simulink model "ES005A_TmplMonr"  (R2013b)
settings: Solver=FixedStepDiscrete  SolverMode=SingleTasking  StartTime=0.0  StopTime=1  FixedStep=0.002  RelTol=1e-3
undefined symbols (not defined in the file): ELECGLBPRM_STRTUPSTDI_CNT_U08, ELECGLBPRM_STRTUPSTTMPLMONININTESTSTRT_CNT_U08, IninFlt, RtFlt, SpiConf_SpiChannel_TmplMonrCh1, SpiConf_SpiChannel_TmplMonrCh2, SpiConf_SpiChannel_TmplMonrCh3, SpiConf_SpiSequence_TmplMonrSeq1, SpiConf_SpiSequence_TmplMonrSeq2, SpiConf_SpiSequence_TmplMonrSeq3, STD_HIGH, STD_LOW, TMPLMONRCFGREG1READVAL_CNT_U16, TMPLMONRCFGREG1WRVAL_CNT_U16, TMPLMONRSTSREG2READVAL_CNT_U16, TMPLMONRWDGMODKEYWORD1_CNT_U16, TMPLMONRWDGMODKEYWORD2_CNT_U16, TMPLMONRWDGMODKEYWORD3_CNT_U16, TrigReg1
libraries: simulink x12
(part 2 of 4)

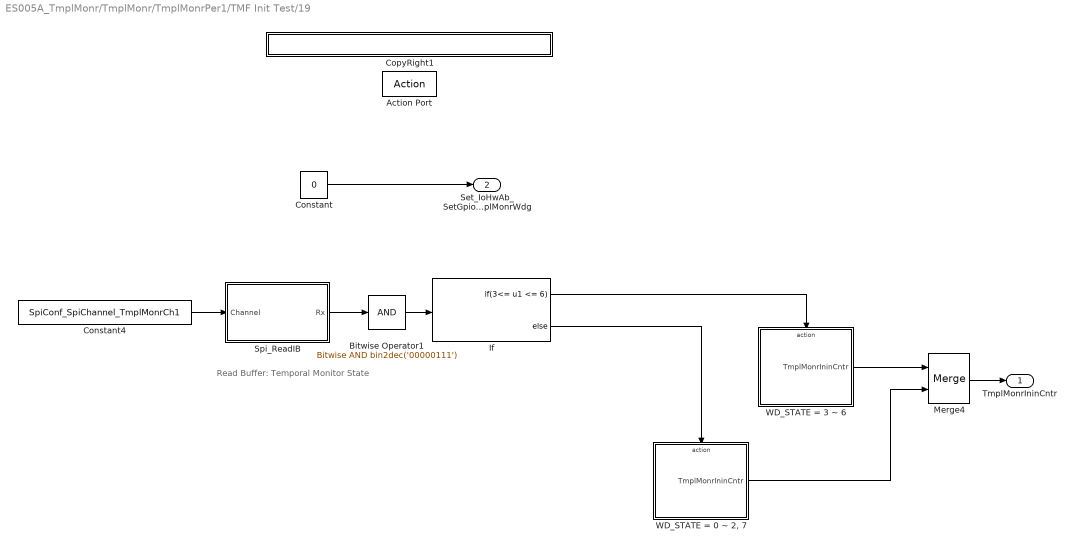
== system ES005A_TmplMonr/TmplMonr/TmplMonrPer1/TMF Init Test/19 ==
  note: Read Buffer: Temporal Monitor State
  Action Port : ActionPort  ActionType=case
  Bitwise Operator1 : simulink/Logic and Bit Operations/Bitwise Operator  logicop=AND  UseBitMask=on  BitMask=bin2dec('00000111')  BitMaskRealWorld=Stored Integer
  Constant : Constant  Value=0  OutDataTypeStr=boolean
  Constant4 : Constant  Value=SpiConf_SpiChannel_TmplMonrCh1  OutDataTypeStr=uint8
  CopyRight1 : Subsystem  Description=|  mask(Copyright Information){none=on}
      | Copyright info block.                                               
      |                                                                     
      | Place copyright information at the top of every subsystem in design.
      mask prompts: none "No parameters"
      mask help: Place copyright information at the top of every subsystem in design.
      mask Display:
      | NxtrConf = 'Nexteer Confidential';
      | 
      | sys = bdroot; %handle for the current model ("system")
      | first = get_param(sys,'Created');
      | first = first(end-3:end);  %year is last four digits
      | 
      | last = get_param(sys,'LastModifiedDate');
      | if isempty(last)
      |     last = datestr(now,'yyyy');
      | else
      |     last = last(end-3:end);
      | end
      | 
      | if strcmp(first,last)
      |     fprintf('%s -- Copyright %s Nexteer',NxtrConf,first)
      | else
      |     fprintf('%s -- %s%s- %s Nexteer',NxtrConf,char(169),first,last)
      | end
  If : If  IfExpression=3<= u1 <= 6
  Merge4 : Merge
  Spi_ReadIB : Subsystem
  "WD_STATE = 0 ~ 2, 7" : Subsystem  RequirementInfo="{'linktype_rmi_doors' '0000c46a (/ESG Group/FDD Module Requirements/EA4 Specific/ES005A_TmplMonr)' '#ES005A_177' 'true' 'REQ: ES005A_177' '' ; 'linktype_rmi_doors' '0000c46a (/ESG Group/FDD Module Requirements/EA4 Specific/ES005A_TmplMonr)' '#ES005A_182' 'true' 'REQ:  ES005A_182' '' } %GIDa_08cc5124_a215_4196_a476_7ca0c813cfd0"
  WD_STATE = 3 ~ 6 : Subsystem
  TmplMonrIninCntr : Outport
  Set_IoHwAb_SetGpioTmplMonrWdg : Outport  Port=2
  wires:
  Bitwise Operator1/1 -> If/1
  If/1 -> WD_STATE = 3 ~ 6/Action
  Constant4/1 -> Spi_ReadIB/1(Channel)
  Spi_ReadIB/1(Rx) -> Bitwise Operator1/1
  If/2 -> "WD_STATE = 0 ~ 2, 7"/Action
  Constant/1 -> Set_IoHwAb_SetGpioTmplMonrWdg/1
  WD_STATE = 3 ~ 6/1(TmplMonrIninCntr) -> Merge4/1
  "WD_STATE = 0 ~ 2, 7"/1(TmplMonrIninCntr) -> Merge4/2
  Merge4/1 -> TmplMonrIninCntr/1

== system ES005A_TmplMonr/TmplMonr/TmplMonrPer1/TMF Init Test/20 ==
  note: 1
  note: Read Cmd: Edge, Valid - 10010000000000
  Action Port : ActionPort  ActionType=case
  Call_Spi_AsyncTransmit : Subsystem
  Constant : Constant  Value=0  OutDataTypeStr=boolean
  Constant2 : Constant  OutDataTypeStr=uint8
  Constant4 : Constant  Value=SpiConf_SpiSequence_TmplMonrSeq3  OutDataTypeStr=uint8
  Constant5 : Constant  Value=SpiConf_SpiChannel_TmplMonrCh3  OutDataTypeStr=uint8
  Constant6 : Constant  Value=TMPLMONRCFGREG1READVAL_CNT_U16  OutDataTypeStr=uint16
  CopyRight1 : Subsystem  Description=|  mask(Copyright Information){none=on}
      | Copyright info block.                                               
      |                                                                     
      | Place copyright information at the top of every subsystem in design.
      mask prompts: none "No parameters"
      mask help: Place copyright information at the top of every subsystem in design.
      mask Display:
      | NxtrConf = 'Nexteer Confidential';
      | 
      | sys = bdroot; %handle for the current model ("system")
      | first = get_param(sys,'Created');
      | first = first(end-3:end);  %year is last four digits
      | 
      | last = get_param(sys,'LastModifiedDate');
      | if isempty(last)
      |     last = datestr(now,'yyyy');
      | else
      |     last = last(end-3:end);
      | end
      | 
      | if strcmp(first,last)
      |     fprintf('%s -- Copyright %s Nexteer',NxtrConf,first)
      | else
      |     fprintf('%s -- %s%s- %s Nexteer',NxtrConf,char(169),first,last)
      | end
  Spi_WriteIB : Subsystem
  TmplMonrIninCntr : Outport
  Set_IoHwAb_SetGpioTmplMonrWdg : Outport  Port=2
  wires:
  Constant2/1 -> TmplMonrIninCntr/1
  Constant4/1 -> Call_Spi_AsyncTransmit/1(Sequence)
  Constant5/1 -> Spi_WriteIB/1(Channel)
  Constant6/1 -> Spi_WriteIB/2(DataBufferPtr)
  Constant/1 -> Set_IoHwAb_SetGpioTmplMonrWdg/1

== system ES005A_TmplMonr/TmplMonr/TmplMonrPer1/TMF Init Test/21 ==
  note: In normal condition the value should be
      | BIN=1011 DEC=11
  note: Read Buffer: Edge/Valid
  Action Port : ActionPort  ActionType=case
  Bitwise Operator1 : simulink/Logic and Bit Operations/Bitwise Operator  logicop=AND  UseBitMask=on  BitMask=bin2dec('00001111')  BitMaskRealWorld=Stored Integer
  Constant : Constant  Value=0  OutDataTypeStr=boolean
  Constant2 : Constant  OutDataTypeStr=uint8
  Constant4 : Constant  Value=SpiConf_SpiChannel_TmplMonrCh3  OutDataTypeStr=uint8
  CopyRight1 : Subsystem  Description=|  mask(Copyright Information){none=on}
      | Copyright info block.                                               
      |                                                                     
      | Place copyright information at the top of every subsystem in design.
      mask prompts: none "No parameters"
      mask help: Place copyright information at the top of every subsystem in design.
      mask Display:
      | NxtrConf = 'Nexteer Confidential';
      | 
      | sys = bdroot; %handle for the current model ("system")
      | first = get_param(sys,'Created');
      | first = first(end-3:end);  %year is last four digits
      | 
      | last = get_param(sys,'LastModifiedDate');
      | if isempty(last)
      |     last = datestr(now,'yyyy');
      | else
      |     last = last(end-3:end);
      | end
      | 
      | if strcmp(first,last)
      |     fprintf('%s -- Copyright %s Nexteer',NxtrConf,first)
      | else
      |     fprintf('%s -- %s%s- %s Nexteer',NxtrConf,char(169),first,last)
      | end
  Edge/Valid Cnts are NOT Correct : Subsystem  RequirementInfo={'linktype_rmi_doors' '0000c46a (/ESG Group/FDD Module Requirements/EA4 Specific/ES005A_TmplMonr)' '#ES005A_176' 'true' 'REQ: ES005A_176' '' } %GIDa_dd7b43f1_2995_4ab0_82fe_3b40abf5c3b8
  If : If  IfExpression=u1 ~= 11  ShowElse=off
  Spi_ReadIB : Subsystem
  TmplMonrIninCntr : Outport
  Set_IoHwAb_SetGpioTmplMonrWdg : Outport  Port=2
  wires:
  Constant4/1 -> Spi_ReadIB/1(Channel)
  Spi_ReadIB/1(Rx) -> Bitwise Operator1/1
  Bitwise Operator1/1 -> If/1
  If/1 -> Edge/Valid Cnts are NOT Correct/Action
  Constant/1 -> Set_IoHwAb_SetGpioTmplMonrWdg/1
  Constant2/1 -> TmplMonrIninCntr/1

== system ES005A_TmplMonr/TmplMonr/TmplMonrPer1/TMF Init Test/22-52 ==
  Action Port : ActionPort  ActionType=case
  Constant : Constant  OutDataTypeStr=boolean
  Constant2 : Constant  OutDataTypeStr=uint8
  CopyRight1 : Subsystem  Description=|  mask(Copyright Information){none=on}
      | Copyright info block.                                               
      |                                                                     
      | Place copyright information at the top of every subsystem in design.
      mask prompts: none "No parameters"
      mask help: Place copyright information at the top of every subsystem in design.
      mask Display:
      | NxtrConf = 'Nexteer Confidential';
      | 
      | sys = bdroot; %handle for the current model ("system")
      | first = get_param(sys,'Created');
      | first = first(end-3:end);  %year is last four digits
      | 
      | last = get_param(sys,'LastModifiedDate');
      | if isempty(last)
      |     last = datestr(now,'yyyy');
      | else
      |     last = last(end-3:end);
      | end
      | 
      | if strcmp(first,last)
      |     fprintf('%s -- Copyright %s Nexteer',NxtrConf,first)
      | else
      |     fprintf('%s -- %s%s- %s Nexteer',NxtrConf,char(169),first,last)
      | end
  TmplMonrIninCntr : Outport
  Set_IoHwAb_SetGpioTmplMonrWdg : Outport  Port=2
  wires:
  Constant2/1 -> TmplMonrIninCntr/1
  Constant/1 -> Set_IoHwAb_SetGpioTmplMonrWdg/1

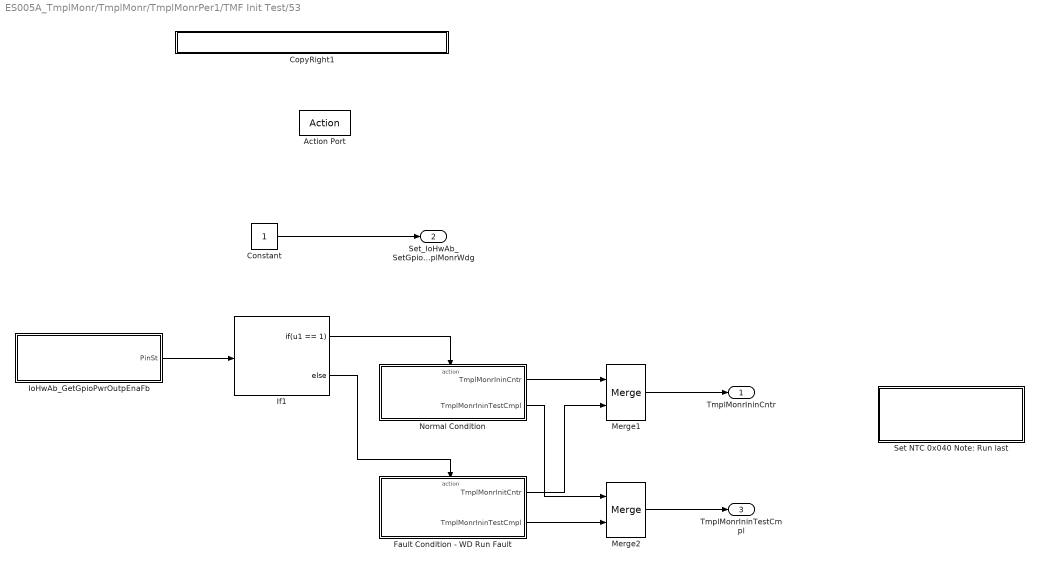
== system ES005A_TmplMonr/TmplMonr/TmplMonrPer1/TMF Init Test/53 ==
  Action Port : ActionPort  ActionType=case
  Constant : Constant  OutDataTypeStr=boolean
  CopyRight1 : Subsystem  Description=|  mask(Copyright Information){none=on}
      | Copyright info block.                                               
      |                                                                     
      | Place copyright information at the top of every subsystem in design.
      mask prompts: none "No parameters"
      mask help: Place copyright information at the top of every subsystem in design.
      mask Display:
      | NxtrConf = 'Nexteer Confidential';
      | 
      | sys = bdroot; %handle for the current model ("system")
      | first = get_param(sys,'Created');
      | first = first(end-3:end);  %year is last four digits
      | 
      | last = get_param(sys,'LastModifiedDate');
      | if isempty(last)
      |     last = datestr(now,'yyyy');
      | else
      |     last = last(end-3:end);
      | end
      | 
      | if strcmp(first,last)
      |     fprintf('%s -- Copyright %s Nexteer',NxtrConf,first)
      | else
      |     fprintf('%s -- %s%s- %s Nexteer',NxtrConf,char(169),first,last)
      | end
  Fault Condition - WD Run Fault : Subsystem  RequirementInfo={} %GIDa_b93698f8_2763_40bb_9d1b_225acd7973d3
  If1 : If  IfExpression=u1 == 1
  IoHwAb_GetGpioPwrOutpEnaFb : Subsystem
  Merge1 : Merge
  Merge2 : Merge
  Normal Condition : Subsystem  RequirementInfo={'linktype_rmi_doors' '0000c46a (/ESG Group/FDD Module Requirements/EA4 Specific/ES005A_TmplMonr)' '#ES005A_164' 'true' 'REQ: ES005A_164' '' } %GIDa_785a744b_ba8b_461e_b98b_5c61c0bc0772
  Set NTC 0x040 Note: Run last : Subsystem  RequirementInfo="{'linktype_rmi_doors' '0000c46a (/ESG Group/FDD Module Requirements/EA4 Specific/ES005A_TmplMonr)' '#ES005A_183' 'true' 'REQ:  ES005A_183' '' } %GIDa_d81dec6a_41a1_4ea0_a985_1fcdbb0d2b96"
  TmplMonrIninCntr : Outport
  Set_IoHwAb_SetGpioTmplMonrWdg : Outport  Port=2
  TmplMonrIninTestCmpl : Outport  Port=3
  wires:
  If1/1 -> Normal Condition/Action
  If1/2 -> Fault Condition - WD Run Fault/Action
  IoHwAb_GetGpioPwrOutpEnaFb/1(PinSt) -> If1/1
  Normal Condition/1(TmplMonrIninCntr) -> Merge1/1
  Fault Condition - WD Run Fault/1(TmplMonrInitCntr) -> Merge1/2
  Constant/1 -> Set_IoHwAb_SetGpioTmplMonrWdg/1
  Merge1/1 -> TmplMonrIninCntr/1
  Merge2/1 -> TmplMonrIninTestCmpl/1
  Normal Condition/2(TmplMonrIninTestCmpl) -> Merge2/1
  Fault Condition - WD Run Fault/2(TmplMonrIninTestCmpl) -> Merge2/2

== system ES005A_TmplMonr/TmplMonr/TmplMonrPer1/TMF Init Test/CopyRight1 ==

== system ES005A_TmplMonr/TmplMonr/TmplMonrPer1/TMF Init Test/Default ==
  note: DO NOTHING
  Action Port : ActionPort  ActionType=default
  CopyRight1 : Subsystem  Description=|  mask(Copyright Information){none=on}
      | Copyright info block.                                               
      |                                                                     
      | Place copyright information at the top of every subsystem in design.
      mask prompts: none "No parameters"
      mask help: Place copyright information at the top of every subsystem in design.
      mask Display:
      | NxtrConf = 'Nexteer Confidential';
      | 
      | sys = bdroot; %handle for the current model ("system")
      | first = get_param(sys,'Created');
      | first = first(end-3:end);  %year is last four digits
      | 
      | last = get_param(sys,'LastModifiedDate');
      | if isempty(last)
      |     last = datestr(now,'yyyy');
      | else
      |     last = last(end-3:end);
      | end
      | 
      | if strcmp(first,last)
      |     fprintf('%s -- Copyright %s Nexteer',NxtrConf,first)
      | else
      |     fprintf('%s -- %s%s- %s Nexteer',NxtrConf,char(169),first,last)
      | end

== system ES005A_TmplMonr/TmplMonr/TmplMonrPer1/TMF Init Test/IoHwAb_SetGpioTmplMonrWdg ==
  Trigger : TriggerPort  PortDimensions=1
  Constant1 : Constant  OutDataTypeStr=boolean
  CopyRight1 : Subsystem  Description=|  mask(Copyright Information){none=on}
      | Copyright info block.                                               
      |                                                                     
      | Place copyright information at the top of every subsystem in design.
      mask prompts: none "No parameters"
      mask help: Place copyright information at the top of every subsystem in design.
      mask Display:
      | NxtrConf = 'Nexteer Confidential';
      | 
      | sys = bdroot; %handle for the current model ("system")
      | first = get_param(sys,'Created');
      | first = first(end-3:end);  %year is last four digits
      | 
      | last = get_param(sys,'LastModifiedDate');
      | if isempty(last)
      |     last = datestr(now,'yyyy');
      | else
      |     last = last(end-3:end);
      | end
      | 
      | if strcmp(first,last)
      |     fprintf('%s -- Copyright %s Nexteer',NxtrConf,first)
      | else
      |     fprintf('%s -- %s%s- %s Nexteer',NxtrConf,char(169),first,last)
      | end
  IoHwAb_SetGpioTmplMonrWdg : Subsystem
  wires:
  Constant1/1 -> IoHwAb_SetGpioTmplMonrWdg/1(PinSt)

== system ES005A_TmplMonr/TmplMonr/TmplMonrPer1/TMF Init Test/nError Signal Control ==
  NerrSt : Inport  RequirementInfo={} %GIDa_e0111a0c_ce8f_4caa_a82b_fb1ad2110f0d
  CopyRight1 : Subsystem  Description=|  mask(Copyright Information){none=on}
      | Copyright info block.                                               
      |                                                                     
      | Place copyright information at the top of every subsystem in design.
      mask prompts: none "No parameters"
      mask help: Place copyright information at the top of every subsystem in design.
      mask Display:
      | NxtrConf = 'Nexteer Confidential';
      | 
      | sys = bdroot; %handle for the current model ("system")
      | first = get_param(sys,'Created');
      | first = first(end-3:end);  %year is last four digits
      | 
      | last = get_param(sys,'LastModifiedDate');
      | if isempty(last)
      |     last = datestr(now,'yyyy');
      | else
      |     last = last(end-3:end);
      | end
      | 
      | if strcmp(first,last)
      |     fprintf('%s -- Copyright %s Nexteer',NxtrConf,first)
      | else
      |     fprintf('%s -- %s%s- %s Nexteer',NxtrConf,char(169),first,last)
      | end
  "CtrlErrOut " : Subsystem
  NtcNr2 : simulink/Sources/Enumerated Constant  OutDataTypeStr=Enum: TrigReg1  Value=TrigReg1.TRIGREG_MSTANDCHKR  SampleTime=inf
  wires:
  NerrSt/1 -> "CtrlErrOut "/1(PinSt_ArgIn)
  NtcNr2/1 -> "CtrlErrOut "/2(TrigReg_ArgIn)

== system ES005A_TmplMonr/TmplMonr/TmplMonrPer1/TMF Run/CopyRight1 ==

== system ES005A_TmplMonr/TmplMonr/TmplMonrPer1/TMF Run/Fault Condition - WD Run Fault ==
  Action Port : ActionPort  ActionType=else
  CopyRight1 : Subsystem  Description=|  mask(Copyright Information){none=on}
      | Copyright info block.                                               
      |                                                                     
      | Place copyright information at the top of every subsystem in design.
      mask prompts: none "No parameters"
      mask help: Place copyright information at the top of every subsystem in design.
      mask Display:
      | NxtrConf = 'Nexteer Confidential';
      | 
      | sys = bdroot; %handle for the current model ("system")
      | first = get_param(sys,'Created');
      | first = first(end-3:end);  %year is last four digits
      | 
      | last = get_param(sys,'LastModifiedDate');
      | if isempty(last)
      |     last = datestr(now,'yyyy');
      | else
      |     last = last(end-3:end);
      | end
      | 
      | if strcmp(first,last)
      |     fprintf('%s -- Copyright %s Nexteer',NxtrConf,first)
      | else
      |     fprintf('%s -- %s%s- %s Nexteer',NxtrConf,char(169),first,last)
      | end
  Data Store Read1 : DataStoreRead  DataStoreName=TmplMonrSpiReadWrOrderFlg2
  If : If  IfExpression=u1 == 0
  "TmplMonrSpiReadWrOrderFlg2 = 0 (Read Cmd) " : Subsystem
  TmplMonrSpiReadWrOrderFlg2 = 1 (Read Buffer) : Subsystem
  wires:
  If/1 -> "TmplMonrSpiReadWrOrderFlg2 = 0 (Read Cmd) "/Action
  If/2 -> TmplMonrSpiReadWrOrderFlg2 = 1 (Read Buffer)/Action
  Data Store Read1/1 -> If/1

== system ES005A_TmplMonr/TmplMonr/TmplMonrPer1/TMF Run/IoHwAb_GetGpioPwrOutpEnaFb ==
  CopyRight1 : Subsystem  Description=|  mask(Copyright Information){none=on}
      | Copyright info block.                                               
      |                                                                     
      | Place copyright information at the top of every subsystem in design.
      mask prompts: none "No parameters"
      mask help: Place copyright information at the top of every subsystem in design.
      mask Display:
      | NxtrConf = 'Nexteer Confidential';
      | 
      | sys = bdroot; %handle for the current model ("system")
      | first = get_param(sys,'Created');
      | first = first(end-3:end);  %year is last four digits
      | 
      | last = get_param(sys,'LastModifiedDate');
      | if isempty(last)
      |     last = datestr(now,'yyyy');
      | else
      |     last = last(end-3:end);
      | end
      | 
      | if strcmp(first,last)
      |     fprintf('%s -- Copyright %s Nexteer',NxtrConf,first)
      | else
      |     fprintf('%s -- %s%s- %s Nexteer',NxtrConf,char(169),first,last)
      | end
  Ground : Ground
  PinSt : Outport
  wires:
  Ground/1 -> PinSt/1

== system ES005A_TmplMonr/TmplMonr/TmplMonrPer1/TMF Run/IoHwAb_SetGpioTmplMonrWdg1 ==
  PinSt : Inport
  CopyRight1 : Subsystem  Description=|  mask(Copyright Information){none=on}
      | Copyright info block.                                               
      |                                                                     
      | Place copyright information at the top of every subsystem in design.
      mask prompts: none "No parameters"
      mask help: Place copyright information at the top of every subsystem in design.
      mask Display:
      | NxtrConf = 'Nexteer Confidential';
      | 
      | sys = bdroot; %handle for the current model ("system")
      | first = get_param(sys,'Created');
      | first = first(end-3:end);  %year is last four digits
      | 
      | last = get_param(sys,'LastModifiedDate');
      | if isempty(last)
      |     last = datestr(now,'yyyy');
      | else
      |     last = last(end-3:end);
      | end
      | 
      | if strcmp(first,last)
      |     fprintf('%s -- Copyright %s Nexteer',NxtrConf,first)
      | else
      |     fprintf('%s -- %s%s- %s Nexteer',NxtrConf,char(169),first,last)
      | end
  Terminator : Terminator
  wires:
  PinSt/1 -> Terminator/1

== system ES005A_TmplMonr/TmplMonr/TmplMonrPer1/TMF Run/Normal Condition ==
  Action Port : ActionPort  ActionType=then
  Constant1 : Constant  Value=0  OutDataTypeStr=boolean
  CopyRight1 : Subsystem  Description=|  mask(Copyright Information){none=on}
      | Copyright info block.                                               
      |                                                                     
      | Place copyright information at the top of every subsystem in design.
      mask prompts: none "No parameters"
      mask help: Place copyright information at the top of every subsystem in design.
      mask Display:
      | NxtrConf = 'Nexteer Confidential';
      | 
      | sys = bdroot; %handle for the current model ("system")
      | first = get_param(sys,'Created');
      | first = first(end-3:end);  %year is last four digits
      | 
      | last = get_param(sys,'LastModifiedDate');
      | if isempty(last)
      |     last = datestr(now,'yyyy');
      | else
      |     last = last(end-3:end);
      | end
      | 
      | if strcmp(first,last)
      |     fprintf('%s -- Copyright %s Nexteer',NxtrConf,first)
      | else
      |     fprintf('%s -- %s%s- %s Nexteer',NxtrConf,char(169),first,last)
      | end
  Data Store Write : DataStoreWrite  DataStoreName=TmplMonrSpiReadWrOrderFlg2
  NtcNr1 : Constant  Value=RtFlt
  NtcStInfo : Constant  Value=0  OutDataTypeStr=uint8
  NtcSts : Constant  Value=0  OutDataTypeStr=uint8
  SetNtcSts : Subsystem
  non debounce : Constant  Value=0  OutDataTypeStr=uint16
  wires:
  NtcNr1/1 -> SetNtcSts/1(NtcNr)
  non debounce/1 -> SetNtcSts/4(DebStep)
  NtcSts/1 -> SetNtcSts/3(NtcSts)
  NtcStInfo/1 -> SetNtcSts/2(NtcStInfo)
  Constant1/1 -> Data Store Write/1

== system ES005A_TmplMonr/TmplMonr/TmplMonrPer2/Subsystem/CopyRight1 ==

== system ES005A_TmplMonr/TmplMonr/TmplMonrPer2/Subsystem/IoHwAb_SetGpioSysFlt2A ==
  PinSt : Inport
  CopyRight1 : Subsystem  Description=|  mask(Copyright Information){none=on}
      | Copyright info block.                                               
      |                                                                     
      | Place copyright information at the top of every subsystem in design.
      mask prompts: none "No parameters"
      mask help: Place copyright information at the top of every subsystem in design.
      mask Display:
      | NxtrConf = 'Nexteer Confidential';
      | 
      | sys = bdroot; %handle for the current model ("system")
      | first = get_param(sys,'Created');
      | first = first(end-3:end);  %year is last four digits
      | 
      | last = get_param(sys,'LastModifiedDate');
      | if isempty(last)
      |     last = datestr(now,'yyyy');
      | else
      |     last = last(end-3:end);
      | end
      | 
      | if strcmp(first,last)
      |     fprintf('%s -- Copyright %s Nexteer',NxtrConf,first)
      | else
      |     fprintf('%s -- %s%s- %s Nexteer',NxtrConf,char(169),first,last)
      | end
  Terminator : Terminator
  wires:
  PinSt/1 -> Terminator/1

== system ES005A_TmplMonr/TmplMonr/TmplMonrPer2/Subsystem/IoHwAb_SetGpioSysFlt2B ==
  PinSt : Inport
  CopyRight1 : Subsystem  Description=|  mask(Copyright Information){none=on}
      | Copyright info block.                                               
      |                                                                     
      | Place copyright information at the top of every subsystem in design.
      mask prompts: none "No parameters"
      mask help: Place copyright information at the top of every subsystem in design.
      mask Display:
      | NxtrConf = 'Nexteer Confidential';
      | 
      | sys = bdroot; %handle for the current model ("system")
      | first = get_param(sys,'Created');
      | first = first(end-3:end);  %year is last four digits
      | 
      | last = get_param(sys,'LastModifiedDate');
      | if isempty(last)
      |     last = datestr(now,'yyyy');
      | else
      |     last = last(end-3:end);
      | end
      | 
      | if strcmp(first,last)
      |     fprintf('%s -- Copyright %s Nexteer',NxtrConf,first)
      | else
      |     fprintf('%s -- %s%s- %s Nexteer',NxtrConf,char(169),first,last)
      | end
  Terminator : Terminator
  wires:
  PinSt/1 -> Terminator/1

== system ES005A_TmplMonr/TmplMonr/TmplMonrPer1/TMF Init Test/0/CopyRight1 ==

== system ES005A_TmplMonr/TmplMonr/TmplMonrPer1/TMF Init Test/0/Watchdog Mode Key: Word1 ==
  note: Write Cmd: Watchdog Mode Key to RESTART - 1111011010011
      | Word1 = 0XD3
  Call_Spi_AsyncTransmit : Subsystem
  Constant1 : Constant  Value=SpiConf_SpiSequence_TmplMonrSeq1  OutDataTypeStr=uint8
  Constant4 : Constant  Value=SpiConf_SpiChannel_TmplMonrCh1  OutDataTypeStr=uint8
  Constant5 : Constant  Value=TMPLMONRWDGMODKEYWORD1_CNT_U16  OutDataTypeStr=uint16
  CopyRight1 : Subsystem  Description=|  mask(Copyright Information){none=on}
      | Copyright info block.                                               
      |                                                                     
      | Place copyright information at the top of every subsystem in design.
      mask prompts: none "No parameters"
      mask help: Place copyright information at the top of every subsystem in design.
      mask Display:
      | NxtrConf = 'Nexteer Confidential';
      | 
      | sys = bdroot; %handle for the current model ("system")
      | first = get_param(sys,'Created');
      | first = first(end-3:end);  %year is last four digits
      | 
      | last = get_param(sys,'LastModifiedDate');
      | if isempty(last)
      |     last = datestr(now,'yyyy');
      | else
      |     last = last(end-3:end);
      | end
      | 
      | if strcmp(first,last)
      |     fprintf('%s -- Copyright %s Nexteer',NxtrConf,first)
      | else
      |     fprintf('%s -- %s%s- %s Nexteer',NxtrConf,char(169),first,last)
      | end
  Spi_WriteIB : Subsystem
  wires:
  Constant1/1 -> Call_Spi_AsyncTransmit/1(Sequence)
  Constant4/1 -> Spi_WriteIB/1(Channel)
  Constant5/1 -> Spi_WriteIB/2(DataBufferPtr)

== system ES005A_TmplMonr/TmplMonr/TmplMonrPer1/TMF Init Test/0/Watchdog Mode Key: Word2 ==
  note: Write Cmd: Watchdog Mode Key to RESTART - 1111000110011
      | Word1 = 0X33
  Call_Spi_AsyncTransmit : Subsystem
  Constant1 : Constant  Value=SpiConf_SpiSequence_TmplMonrSeq2  OutDataTypeStr=uint8
  Constant4 : Constant  Value=SpiConf_SpiChannel_TmplMonrCh2  OutDataTypeStr=uint8
  Constant5 : Constant  Value=TMPLMONRWDGMODKEYWORD2_CNT_U16  OutDataTypeStr=uint16
  CopyRight1 : Subsystem  Description=|  mask(Copyright Information){none=on}
      | Copyright info block.                                               
      |                                                                     
      | Place copyright information at the top of every subsystem in design.
      mask prompts: none "No parameters"
      mask help: Place copyright information at the top of every subsystem in design.
      mask Display:
      | NxtrConf = 'Nexteer Confidential';
      | 
      | sys = bdroot; %handle for the current model ("system")
      | first = get_param(sys,'Created');
      | first = first(end-3:end);  %year is last four digits
      | 
      | last = get_param(sys,'LastModifiedDate');
      | if isempty(last)
      |     last = datestr(now,'yyyy');
      | else
      |     last = last(end-3:end);
      | end
      | 
      | if strcmp(first,last)
      |     fprintf('%s -- Copyright %s Nexteer',NxtrConf,first)
      | else
      |     fprintf('%s -- %s%s- %s Nexteer',NxtrConf,char(169),first,last)
      | end
  Spi_WriteIB : Subsystem
  wires:
  Constant5/1 -> Spi_WriteIB/2(DataBufferPtr)
  Constant4/1 -> Spi_WriteIB/1(Channel)
  Constant1/1 -> Call_Spi_AsyncTransmit/1(Sequence)

== system ES005A_TmplMonr/TmplMonr/TmplMonrPer1/TMF Init Test/0/Watchdog Mode Key: Word3 ==
  note: Write Cmd: Watchdog Mode Key to RESTART - 1111011001101
      | Word1 = 0XCD
  Call_Spi_AsyncTransmit : Subsystem
  Constant1 : Constant  Value=SpiConf_SpiSequence_TmplMonrSeq3  OutDataTypeStr=uint8
  Constant4 : Constant  Value=SpiConf_SpiChannel_TmplMonrCh3  OutDataTypeStr=uint8
  Constant5 : Constant  Value=TMPLMONRWDGMODKEYWORD3_CNT_U16  OutDataTypeStr=uint16
  CopyRight1 : Subsystem  Description=|  mask(Copyright Information){none=on}
      | Copyright info block.                                               
      |                                                                     
      | Place copyright information at the top of every subsystem in design.
      mask prompts: none "No parameters"
      mask help: Place copyright information at the top of every subsystem in design.
      mask Display:
      | NxtrConf = 'Nexteer Confidential';
      | 
      | sys = bdroot; %handle for the current model ("system")
      | first = get_param(sys,'Created');
      | first = first(end-3:end);  %year is last four digits
      | 
      | last = get_param(sys,'LastModifiedDate');
      | if isempty(last)
      |     last = datestr(now,'yyyy');
      | else
      |     last = last(end-3:end);
      | end
      | 
      | if strcmp(first,last)
      |     fprintf('%s -- Copyright %s Nexteer',NxtrConf,first)
      | else
      |     fprintf('%s -- %s%s- %s Nexteer',NxtrConf,char(169),first,last)
      | end
  Spi_WriteIB : Subsystem
  wires:
  Constant1/1 -> Call_Spi_AsyncTransmit/1(Sequence)
  Constant4/1 -> Spi_WriteIB/1(Channel)
  Constant5/1 -> Spi_WriteIB/2(DataBufferPtr)

== system ES005A_TmplMonr/TmplMonr/TmplMonrPer1/TMF Init Test/1-9/CopyRight1 ==

== system ES005A_TmplMonr/TmplMonr/TmplMonrPer1/TMF Init Test/10-11, 15-17/CopyRight1 ==

== system ES005A_TmplMonr/TmplMonr/TmplMonrPer1/TMF Init Test/10-11, 15-17/IoHwAb_GetGpioPwrOutpEnaFb1 ==
  Action Port : ActionPort  ActionType=then
  CopyRight1 : Subsystem  Description=|  mask(Copyright Information){none=on}
      | Copyright info block.                                               
      |                                                                     
      | Place copyright information at the top of every subsystem in design.
      mask prompts: none "No parameters"
      mask help: Place copyright information at the top of every subsystem in design.
      mask Display:
      | NxtrConf = 'Nexteer Confidential';
      | 
      | sys = bdroot; %handle for the current model ("system")
      | first = get_param(sys,'Created');
      | first = first(end-3:end);  %year is last four digits
      | 
      | last = get_param(sys,'LastModifiedDate');
      | if isempty(last)
      |     last = datestr(now,'yyyy');
      | else
      |     last = last(end-3:end);
      | end
      | 
      | if strcmp(first,last)
      |     fprintf('%s -- Copyright %s Nexteer',NxtrConf,first)
      | else
      |     fprintf('%s -- %s%s- %s Nexteer',NxtrConf,char(169),first,last)
      | end
  Fault Condition - WD Signal : Subsystem  RequirementInfo={'linktype_rmi_doors' '0000c46a (/ESG Group/FDD Module Requirements/EA4 Specific/ES005A_TmplMonr)' '#ES005A_158' 'true' 'REQ: ES005A_158' '' ; 'linktype_rmi_doors' '0000c46a (/ESG Group/FDD Module Requirements/EA4 Specific/ES005A_TmplMonr)' '#ES005A_163' 'true' 'REQ: ES005A_163' '' ; 'linktype_rmi_doors' '0000c46a (/ESG Group/FDD Module Requirements/EA4 Specific/ES005A_TmplMonr)' '#ES005A_172' 'true' 'REQ: ES005A_172' '' } %GIDa_89a4d9ae_99ea_4011_b803_c994c7645272
  If1 : If  RequirementInfo={'linktype_rmi_doors' '0000c46a (/ESG Group/FDD Module Requirements/EA4 Specific/ES005A_TmplMonr)' '#ES005A_163' 'true' 'REQ: ES005A_163' '' ; 'linktype_rmi_doors' '0000c46a (/ESG Group/FDD Module Requirements/EA4 Specific/ES005A_TmplMonr)' '#ES005A_172' 'true' 'REQ: ES005A_172' '' } %GIDa_4f483320_e134_42eb_ab01_bf1264f50d52  IfExpression=u1 ~= 1  ShowElse=off
  IoHwAb_GetGpioPwrOutpEnaFb : Subsystem
  wires:
  If1/1 -> Fault Condition - WD Signal/Action
  IoHwAb_GetGpioPwrOutpEnaFb/1(PinSt) -> If1/1

== system ES005A_TmplMonr/TmplMonr/TmplMonrPer1/TMF Init Test/12/CopyRight1 ==

== system ES005A_TmplMonr/TmplMonr/TmplMonrPer1/TMF Init Test/13/CopyRight1 ==

== system ES005A_TmplMonr/TmplMonr/TmplMonrPer1/TMF Init Test/13/Fault Condition - AND Gate ==
  note: NTCNR_0X040
      | Parameters:
      |     1 = 0000 0001 = Bit 0 = Fault Occured Between TmplMonrInitCntr =  10 ~ 11
      |     2 = 0000 0010 = Bit 1 = Fault Occured Between TmplMonrInitCntr = 13 (AND Gate Fault)
      |     4 = 0000 0100 = Bit 2 = Fault Occured Between TmplMonrInitCntr = 15 ~ 16
      |     8 = 0000 1000 = Bit 3 = Fault Occured at TmplMonrInitCntr            = 18  (POE Fault)
      |   16 = 0001 0000 = Bit 4 = Fault Occured at TmplMonrInitCntr            = 19 (WD_STATE Fault)
      |   32 = 0010 0000 = Bit 5 = Fault Occured at TmplMonrInitCntr            = 21 (Edge/Valid Write Fault)
      |   64 = 0100 0000 = Bit 6 = Fault Occured at TmplMonrInitCntr            = 53 (POE + Non-WD Fault)
      | 128 = 1000 0000 = Bit 7 = Fault Occured at TmplMonrInitCntr            = 53 (POE + WD Fault)
  Action Port : ActionPort  ActionType=then
  Bitwise Operator2 : simulink/Logic and Bit Operations/Bitwise Operator  logicop=OR  UseBitMask=off  NumInputPorts=2  BitMask=bin2dec('00001111')  BitMaskRealWorld=Stored Integer
  CopyRight1 : Subsystem  Description=|  mask(Copyright Information){none=on}
      | Copyright info block.                                               
      |                                                                     
      | Place copyright information at the top of every subsystem in design.
      mask prompts: none "No parameters"
      mask help: Place copyright information at the top of every subsystem in design.
      mask Display:
      | NxtrConf = 'Nexteer Confidential';
      | 
      | sys = bdroot; %handle for the current model ("system")
      | first = get_param(sys,'Created');
      | first = first(end-3:end);  %year is last four digits
      | 
      | last = get_param(sys,'LastModifiedDate');
      | if isempty(last)
      |     last = datestr(now,'yyyy');
      | else
      |     last = last(end-3:end);
      | end
      | 
      | if strcmp(first,last)
      |     fprintf('%s -- Copyright %s Nexteer',NxtrConf,first)
      | else
      |     fprintf('%s -- %s%s- %s Nexteer',NxtrConf,char(169),first,last)
      | end
  Data Store Read3 : DataStoreRead  DataStoreName=TmplMonrNtc40PrmByte  DataStoreElements=TmplMonrNtc40PrmByte
  Data Store Write1 : DataStoreWrite  DataStoreName=TmplMonrNtc40PrmByte
  NtcStInfo : Constant  Value=2  OutDataTypeStr=uint8
  wires:
  Bitwise Operator2/1 -> Data Store Write1/1
  Data Store Read3/1 -> Bitwise Operator2/1
  NtcStInfo/1 -> Bitwise Operator2/2

== system ES005A_TmplMonr/TmplMonr/TmplMonrPer1/TMF Init Test/13/IoHwAb_GetGpioPwrOutpEnaFb ==
  CopyRight1 : Subsystem  Description=|  mask(Copyright Information){none=on}
      | Copyright info block.                                               
      |                                                                     
      | Place copyright information at the top of every subsystem in design.
      mask prompts: none "No parameters"
      mask help: Place copyright information at the top of every subsystem in design.
      mask Display:
      | NxtrConf = 'Nexteer Confidential';
      | 
      | sys = bdroot; %handle for the current model ("system")
      | first = get_param(sys,'Created');
      | first = first(end-3:end);  %year is last four digits
      | 
      | last = get_param(sys,'LastModifiedDate');
      | if isempty(last)
      |     last = datestr(now,'yyyy');
      | else
      |     last = last(end-3:end);
      | end
      | 
      | if strcmp(first,last)
      |     fprintf('%s -- Copyright %s Nexteer',NxtrConf,first)
      | else
      |     fprintf('%s -- %s%s- %s Nexteer',NxtrConf,char(169),first,last)
      | end
  Ground : Ground
  PinSt : Outport
  wires:
  Ground/1 -> PinSt/1

== system ES005A_TmplMonr/TmplMonr/TmplMonrPer1/TMF Init Test/14/CopyRight1 ==

== system ES005A_TmplMonr/TmplMonr/TmplMonrPer1/TMF Init Test/18/Call_Spi_AsyncTransmit ==
  Sequence : Inport
  CopyRight1 : Subsystem  Description=|  mask(Copyright Information){none=on}
      | Copyright info block.                                               
      |                                                                     
      | Place copyright information at the top of every subsystem in design.
      mask prompts: none "No parameters"
      mask help: Place copyright information at the top of every subsystem in design.
      mask Display:
      | NxtrConf = 'Nexteer Confidential';
      | 
      | sys = bdroot; %handle for the current model ("system")
      | first = get_param(sys,'Created');
      | first = first(end-3:end);  %year is last four digits
      | 
      | last = get_param(sys,'LastModifiedDate');
      | if isempty(last)
      |     last = datestr(now,'yyyy');
      | else
      |     last = last(end-3:end);
      | end
      | 
      | if strcmp(first,last)
      |     fprintf('%s -- Copyright %s Nexteer',NxtrConf,first)
      | else
      |     fprintf('%s -- %s%s- %s Nexteer',NxtrConf,char(169),first,last)
      | end
  Terminator : Terminator
  wires:
  Sequence/1 -> Terminator/1

== system ES005A_TmplMonr/TmplMonr/TmplMonrPer1/TMF Init Test/18/CopyRight1 ==

== system ES005A_TmplMonr/TmplMonr/TmplMonrPer1/TMF Init Test/18/Fault Condition - WD ==
  note: NTCNR_0X040
      | Parameters:
      |     1 = 0000 0001 = Bit 0 = Fault Occured Between TmplMonrInitCntr =  10 ~ 11
      |     2 = 0000 0010 = Bit 1 = Fault Occured Between TmplMonrInitCntr = 13 (AND Gate Fault)
      |     4 = 0000 0100 = Bit 2 = Fault Occured Between TmplMonrInitCntr = 15 ~ 16
      |     8 = 0000 1000 = Bit 3 = Fault Occured at TmplMonrInitCntr            = 18  (POE Fault)
      |   16 = 0001 0000 = Bit 4 = Fault Occured at TmplMonrInitCntr            = 19 (WD_STATE Fault)
      |   32 = 0010 0000 = Bit 5 = Fault Occured at TmplMonrInitCntr            = 21 (Edge/Valid Write Fault)
      |   64 = 0100 0000 = Bit 6 = Fault Occured at TmplMonrInitCntr            = 53 (POE + Non-WD Fault)
      | 128 = 1000 0000 = Bit 7 = Fault Occured at TmplMonrInitCntr            = 53 (POE + WD Fault)
  Action Port : ActionPort  ActionType=then
  Bitwise Operator2 : simulink/Logic and Bit Operations/Bitwise Operator  logicop=OR  UseBitMask=off  NumInputPorts=2  BitMask=bin2dec('00001111')  BitMaskRealWorld=Stored Integer
  CopyRight1 : Subsystem  Description=|  mask(Copyright Information){none=on}
      | Copyright info block.                                               
      |                                                                     
      | Place copyright information at the top of every subsystem in design.
      mask prompts: none "No parameters"
      mask help: Place copyright information at the top of every subsystem in design.
      mask Display:
      | NxtrConf = 'Nexteer Confidential';
      | 
      | sys = bdroot; %handle for the current model ("system")
      | first = get_param(sys,'Created');
      | first = first(end-3:end);  %year is last four digits
      | 
      | last = get_param(sys,'LastModifiedDate');
      | if isempty(last)
      |     last = datestr(now,'yyyy');
      | else
      |     last = last(end-3:end);
      | end
      | 
      | if strcmp(first,last)
      |     fprintf('%s -- Copyright %s Nexteer',NxtrConf,first)
      | else
      |     fprintf('%s -- %s%s- %s Nexteer',NxtrConf,char(169),first,last)
      | end
  Data Store Read3 : DataStoreRead  DataStoreName=TmplMonrNtc40PrmByte  DataStoreElements=TmplMonrNtc40PrmByte
  Data Store Write1 : DataStoreWrite  DataStoreName=TmplMonrNtc40PrmByte
  NtcStInfo : Constant  Value=8  OutDataTypeStr=uint8
  wires:
  Bitwise Operator2/1 -> Data Store Write1/1
  Data Store Read3/1 -> Bitwise Operator2/1
  NtcStInfo/1 -> Bitwise Operator2/2

== system ES005A_TmplMonr/TmplMonr/TmplMonrPer1/TMF Init Test/18/IoHwAb_GetGpioPwrOutpEnaFb ==
  CopyRight1 : Subsystem  Description=|  mask(Copyright Information){none=on}
      | Copyright info block.                                               
      |                                                                     
      | Place copyright information at the top of every subsystem in design.
      mask prompts: none "No parameters"
      mask help: Place copyright information at the top of every subsystem in design.
      mask Display:
      | NxtrConf = 'Nexteer Confidential';
      | 
      | sys = bdroot; %handle for the current model ("system")
      | first = get_param(sys,'Created');
      | first = first(end-3:end);  %year is last four digits
      | 
      | last = get_param(sys,'LastModifiedDate');
      | if isempty(last)
      |     last = datestr(now,'yyyy');
      | else
      |     last = last(end-3:end);
      | end
      | 
      | if strcmp(first,last)
      |     fprintf('%s -- Copyright %s Nexteer',NxtrConf,first)
      | else
      |     fprintf('%s -- %s%s- %s Nexteer',NxtrConf,char(169),first,last)
      | end
  Ground : Ground
  PinSt : Outport
  wires:
  Ground/1 -> PinSt/1

== system ES005A_TmplMonr/TmplMonr/TmplMonrPer1/TMF Init Test/18/Spi_WriteIB ==
  Channel : Inport
  DataBufferPtr : Inport  Port=2
  CopyRight1 : Subsystem  Description=|  mask(Copyright Information){none=on}
      | Copyright info block.                                               
      |                                                                     
      | Place copyright information at the top of every subsystem in design.
      mask prompts: none "No parameters"
      mask help: Place copyright information at the top of every subsystem in design.
      mask Display:
      | NxtrConf = 'Nexteer Confidential';
      | 
      | sys = bdroot; %handle for the current model ("system")
      | first = get_param(sys,'Created');
      | first = first(end-3:end);  %year is last four digits
      | 
      | last = get_param(sys,'LastModifiedDate');
      | if isempty(last)
      |     last = datestr(now,'yyyy');
      | else
      |     last = last(end-3:end);
      | end
      | 
      | if strcmp(first,last)
      |     fprintf('%s -- Copyright %s Nexteer',NxtrConf,first)
      | else
      |     fprintf('%s -- %s%s- %s Nexteer',NxtrConf,char(169),first,last)
      | end
  Terminator : Terminator
  Terminator1 : Terminator
  wires:
  Channel/1 -> Terminator/1
  DataBufferPtr/1 -> Terminator1/1

== system ES005A_TmplMonr/TmplMonr/TmplMonrPer1/TMF Init Test/19/CopyRight1 ==

== system ES005A_TmplMonr/TmplMonr/TmplMonrPer1/TMF Init Test/19/Spi_ReadIB ==
  note: 00101100
  note: Read Buffer - Simulation Purpose Only
  Channel : Inport
  Constant3 : Constant  Value=44  OutDataTypeStr=uint16
  CopyRight1 : Subsystem  Description=|  mask(Copyright Information){none=on}
      | Copyright info block.                                               
      |                                                                     
      | Place copyright information at the top of every subsystem in design.
      mask prompts: none "No parameters"
      mask help: Place copyright information at the top of every subsystem in design.
      mask Display:
      | NxtrConf = 'Nexteer Confidential';
      | 
      | sys = bdroot; %handle for the current model ("system")
      | first = get_param(sys,'Created');
      | first = first(end-3:end);  %year is last four digits
      | 
      | last = get_param(sys,'LastModifiedDate');
      | if isempty(last)
      |     last = datestr(now,'yyyy');
      | else
      |     last = last(end-3:end);
      | end
      | 
      | if strcmp(first,last)
      |     fprintf('%s -- Copyright %s Nexteer',NxtrConf,first)
      | else
      |     fprintf('%s -- %s%s- %s Nexteer',NxtrConf,char(169),first,last)
      | end
  Terminator : Terminator
  Rx : Outport
  wires:
  Constant3/1 -> Rx/1
  Channel/1 -> Terminator/1

== system ES005A_TmplMonr/TmplMonr/TmplMonrPer1/TMF Init Test/19/WD_STATE = 0 ~ 2, 7 ==
  note: NTCNR_0X040
      | Parameters:
      |     1 = 0000 0001 = Bit 0 = Fault Occured Between TmplMonrInitCntr =  10 ~ 11
      |     2 = 0000 0010 = Bit 1 = Fault Occured Between TmplMonrInitCntr = 13 (AND Gate Fault)
      |     4 = 0000 0100 = Bit 2 = Fault Occured Between TmplMonrInitCntr = 15 ~ 16
      |     8 = 0000 1000 = Bit 3 = Fault Occured at TmplMonrInitCntr            = 18  (POE Fault)
      |   16 = 0001 0000 = Bit 4 = Fault Occured at TmplMonrInitCntr            = 19 (WD_STATE Fault)
      |   32 = 0010 0000 = Bit 5 = Fault Occured at TmplMonrInitCntr            = 21 (Edge/Valid Write Fault)
      |   64 = 0100 0000 = Bit 6 = Fault Occured at TmplMonrInitCntr            = 53 (POE + Non-WD Fault)
      | 128 = 1000 0000 = Bit 7 = Fault Occured at TmplMonrInitCntr            = 53 (POE + WD Fault)
  Action Port : ActionPort  ActionType=else
  Constant2 : Constant  Value=0  OutDataTypeStr=uint8
  CopyRight1 : Subsystem  Description=|  mask(Copyright Information){none=on}
      | Copyright info block.                                               
      |                                                                     
      | Place copyright information at the top of every subsystem in design.
      mask prompts: none "No parameters"
      mask help: Place copyright information at the top of every subsystem in design.
      mask Display:
      | NxtrConf = 'Nexteer Confidential';
      | 
      | sys = bdroot; %handle for the current model ("system")
      | first = get_param(sys,'Created');
      | first = first(end-3:end);  %year is last four digits
      | 
      | last = get_param(sys,'LastModifiedDate');
      | if isempty(last)
      |     last = datestr(now,'yyyy');
      | else
      |     last = last(end-3:end);
      | end
      | 
      | if strcmp(first,last)
      |     fprintf('%s -- Copyright %s Nexteer',NxtrConf,first)
      | else
      |     fprintf('%s -- %s%s- %s Nexteer',NxtrConf,char(169),first,last)
      | end
  Data Store Read1 : DataStoreRead  DataStoreName=TmplMonrWdgRstrtCnt
  If : If  IfExpression=u1 <= 1
  Jump to Stage 53 : Subsystem
  WD RESTART - Two Retry : Subsystem
  TmplMonrIninCntr : Outport
  wires:
  If/1 -> WD RESTART - Two Retry/Action
  If/2 -> Jump to Stage 53/Action
  Data Store Read1/1 -> If/1
  Constant2/1 -> TmplMonrIninCntr/1

== system ES005A_TmplMonr/TmplMonr/TmplMonrPer1/TMF Init Test/19/WD_STATE = 3 ~ 6 ==
  note: Write: Edge/Valid - 10011000001011
  Action Port : ActionPort  ActionType=then
  Call_Spi_AsyncTransmit : Subsystem
  Constant1 : Constant  Value=SpiConf_SpiSequence_TmplMonrSeq2  OutDataTypeStr=uint8
  Constant2 : Constant  OutDataTypeStr=uint8
  Constant4 : Constant  Value=SpiConf_SpiChannel_TmplMonrCh2  OutDataTypeStr=uint8
  Constant5 : Constant  Value=TMPLMONRCFGREG1WRVAL_CNT_U16  OutDataTypeStr=uint16
  CopyRight1 : Subsystem  Description=|  mask(Copyright Information){none=on}
      | Copyright info block.                                               
      |                                                                     
      | Place copyright information at the top of every subsystem in design.
      mask prompts: none "No parameters"
      mask help: Place copyright information at the top of every subsystem in design.
      mask Display:
      | NxtrConf = 'Nexteer Confidential';
      | 
      | sys = bdroot; %handle for the current model ("system")
      | first = get_param(sys,'Created');
      | first = first(end-3:end);  %year is last four digits
      | 
      | last = get_param(sys,'LastModifiedDate');
      | if isempty(last)
      |     last = datestr(now,'yyyy');
      | else
      |     last = last(end-3:end);
      | end
      | 
      | if strcmp(first,last)
      |     fprintf('%s -- Copyright %s Nexteer',NxtrConf,first)
      | else
      |     fprintf('%s -- %s%s- %s Nexteer',NxtrConf,char(169),first,last)
      | end
  Spi_WriteIB : Subsystem
  TmplMonrIninCntr : Outport
  wires:
  Constant1/1 -> Call_Spi_AsyncTransmit/1(Sequence)
  Constant4/1 -> Spi_WriteIB/1(Channel)
  Constant5/1 -> Spi_WriteIB/2(DataBufferPtr)
  Constant2/1 -> TmplMonrIninCntr/1

== system ES005A_TmplMonr/TmplMonr/TmplMonrPer1/TMF Init Test/20/Call_Spi_AsyncTransmit ==
  Sequence : Inport
  CopyRight1 : Subsystem  Description=|  mask(Copyright Information){none=on}
      | Copyright info block.                                               
      |                                                                     
      | Place copyright information at the top of every subsystem in design.
      mask prompts: none "No parameters"
      mask help: Place copyright information at the top of every subsystem in design.
      mask Display:
      | NxtrConf = 'Nexteer Confidential';
      | 
      | sys = bdroot; %handle for the current model ("system")
      | first = get_param(sys,'Created');
      | first = first(end-3:end);  %year is last four digits
      | 
      | last = get_param(sys,'LastModifiedDate');
      | if isempty(last)
      |     last = datestr(now,'yyyy');
      | else
      |     last = last(end-3:end);
      | end
      | 
      | if strcmp(first,last)
      |     fprintf('%s -- Copyright %s Nexteer',NxtrConf,first)
      | else
      |     fprintf('%s -- %s%s- %s Nexteer',NxtrConf,char(169),first,last)
      | end
  Terminator : Terminator
  wires:
  Sequence/1 -> Terminator/1

== system ES005A_TmplMonr/TmplMonr/TmplMonrPer1/TMF Init Test/20/CopyRight1 ==

== system ES005A_TmplMonr/TmplMonr/TmplMonrPer1/TMF Init Test/20/Spi_WriteIB ==
  Channel : Inport
  DataBufferPtr : Inport  Port=2
  CopyRight1 : Subsystem  Description=|  mask(Copyright Information){none=on}
      | Copyright info block.                                               
      |                                                                     
      | Place copyright information at the top of every subsystem in design.
      mask prompts: none "No parameters"
      mask help: Place copyright information at the top of every subsystem in design.
      mask Display:
      | NxtrConf = 'Nexteer Confidential';
      | 
      | sys = bdroot; %handle for the current model ("system")
      | first = get_param(sys,'Created');
      | first = first(end-3:end);  %year is last four digits
      | 
      | last = get_param(sys,'LastModifiedDate');
      | if isempty(last)
      |     last = datestr(now,'yyyy');
      | else
      |     last = last(end-3:end);
      | end
      | 
      | if strcmp(first,last)
      |     fprintf('%s -- Copyright %s Nexteer',NxtrConf,first)
      | else
      |     fprintf('%s -- %s%s- %s Nexteer',NxtrConf,char(169),first,last)
      | end
  Terminator : Terminator
  Terminator1 : Terminator
  wires:
  Channel/1 -> Terminator/1
  DataBufferPtr/1 -> Terminator1/1
